simulink model "problem_3"  (R2020a)
settings: Solver=FixedStepAuto  StartTime=0.0  StopTime=120  FixedStep=0.01  RelTol=1e-3
model workspace (MAT data in the model file):
  b = 50
  kd = 0
  ki = 100
  kp = 600
  m = 1000
  u = 500
settings Model: Creator=Shubham Singh Rathor  LastModifiedBy=Shubham Singh Rathor
settings SolverCC: AlgebraicLoopSolver=LineSearch

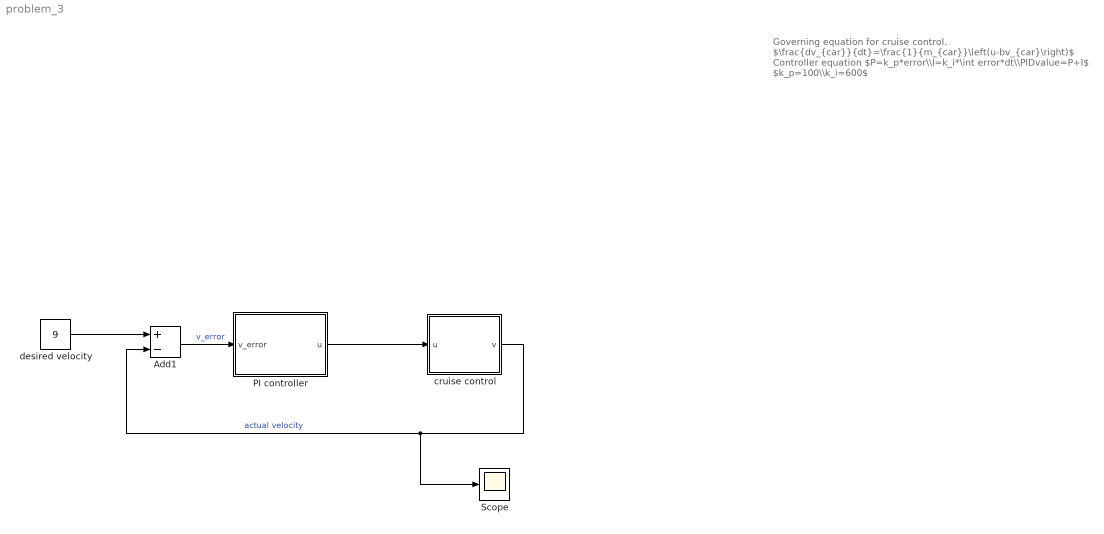
== system problem_3 ==
  note: Governing equation for cruise control.
      | $\frac{dv_{car}}{dt}=\frac{1}{m_{car}}\left(u-bv_{car}\right)$
      |
      | Controller equation
      | $P=k_p*error\\I=k_i*\int error*dt\\PIDvalue=P+I$
      | $k_p=100\\k_i=600$
  Add1 : Sum  Inputs=+-
  PI controller : Subsystem
  Scope : Scope
  cruise control : Subsystem
  desired velocity : Constant  Value=9
  wires:
  desired velocity/1 -> Add1/1
  cruise control/1(v) -> Scope/1, Add1/2  "actual velocity"
  Add1/1 -> PI controller/1(v_error)  "v_error"
  PI controller/1(u) -> cruise control/1(u)

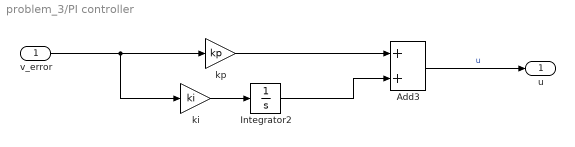
== system problem_3/PI controller ==
  v_error : Inport
  Add3 : Sum
  Integrator2 : Integrator
  ki : Gain  Gain=ki
  kp : Gain  Gain=kp
  u : Outport
  wires:
  kp/1 -> Add3/1
  v_error/1 -> kp/1, ki/1
  Integrator2/1 -> Add3/2
  ki/1 -> Integrator2/1
  Add3/1 -> u/1  "u"

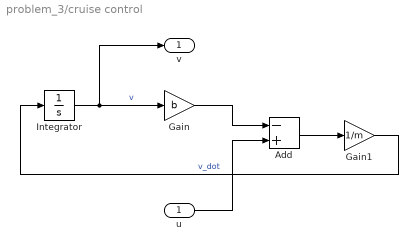
== system problem_3/cruise control ==
  u : Inport
  Add : Sum  Inputs=-+
  Gain : Gain  Gain=b
  Gain1 : Gain  Gain=1/m
  Integrator : Integrator
  v : Outport
  wires:
  Integrator/1 -> v/1, Gain/1  "v"
  Gain/1 -> Add/1
  Gain1/1 -> Integrator/1  "v_dot"
  Add/1 -> Gain1/1
  u/1 -> Add/2
